simulink model "TorqueAchievedEstimationComponent"  (R2026a)
settings: Solver=FixedStepDiscrete
settings Model: DataDictionary=TractionEmotorSoftwareArchInterfaceData.sldd  Creator=dakaihu  LastModifiedBy=dakaihu

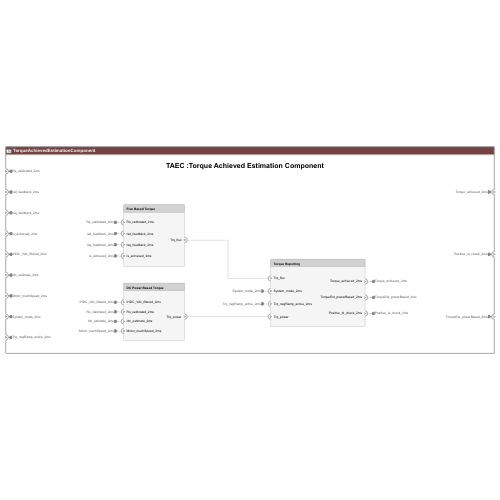
[thumbnail: Simulink's stored preview of the top-level diagram]
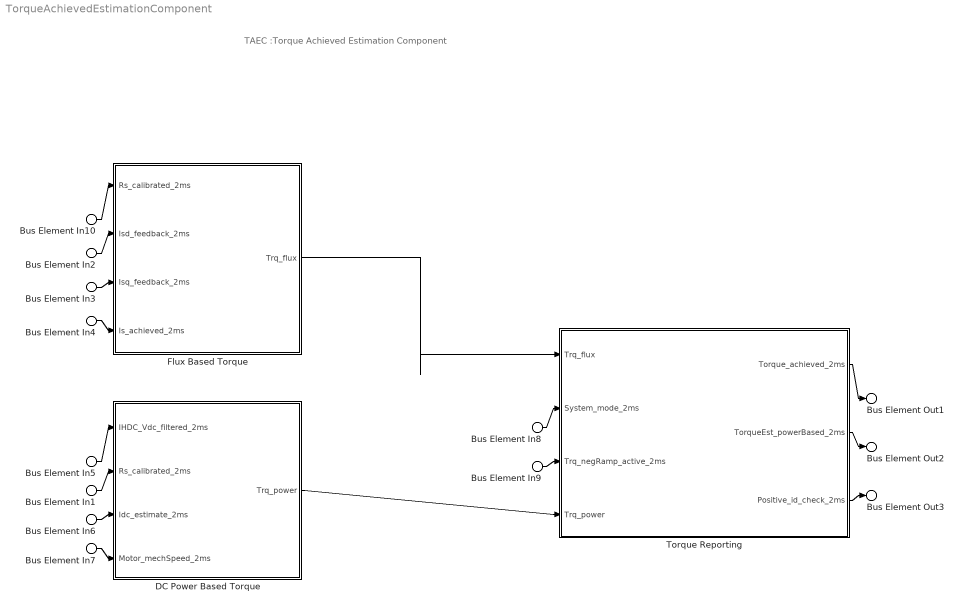
== system TorqueAchievedEstimationComponent ==
  note: TAEC :Torque Achieved Estimation Component
  Bus Element In1 : Inport  PortName=Rs_calibrated_2ms
  Bus Element In10 : Inport  PortName=Rs_calibrated_2ms
  Bus Element In2 : Inport  Port=2  PortName=Isd_feedback_2ms
  Bus Element In3 : Inport  Port=3  PortName=Isq_feedback_2ms
  Bus Element In4 : Inport  Port=4  PortName=Is_achieved_2ms
  Bus Element In5 : Inport  Port=5  PortName=IHDC_Vdc_filtered_2ms
  Bus Element In6 : Inport  Port=6  PortName=Idc_estimate_2ms
  Bus Element In7 : Inport  Port=7  PortName=Motor_mechSpeed_2ms
  Bus Element In8 : Inport  Port=8  PortName=System_mode_2ms
  Bus Element In9 : Inport  Port=9  PortName=Trq_negRamp_active_2ms
  DC Power Based Torque : Subsystem
      settings: PortSchema="{\"entries\":[{\"content\":{\"headerSize\":26,\"margin\":15,\"minimumSpacing\":25,\"sides\":[{\"content\":{\"connectorIds\":[\"In1\",\"In2\",\"In3\",\"In4\"]},\"type\":\"ConnectorPlacement.EquallySpacedRectSide\",\"uuid\":\"a0c63ab2-75fe-4bec-b2b0-6e2e00a1a5a4\"},{\"content\":{\"connectorIds\":[\"Out1\"],\"side\":\"RIGHT\"},\"type\":\"ConnectorPlacement.EquallySpacedRectSide\",\"uuid\":\"05d605ea-8968-4533-a01c-bf4aae5caa93\"},{\"content\":{\"side\":\"TOP\"},\"type\":\"ConnectorPlacement.EquallySpacedRectSide\",\"uuid\":\"27167c69-3967-4107-acce-f317c3d854af\"}]},\"type\":\"ConnectorPlacement.EquallySpacedConnector\",\"uuid\":\"c4d90da2-0f2a-4c00-bd24-85fead00d18f\"}],\"packageUris\":[\"http://schema.mathworks.com/mf0/Connector/R2020b\"],\"version\":\"1.0\"}"
  Flux Based Torque : Subsystem
      settings: PortSchema="{\"entries\":[{\"content\":{\"headerSize\":26,\"margin\":15,\"minimumSpacing\":25,\"sides\":[{\"content\":{\"connectorIds\":[\"In1\",\"In2\",\"In3\",\"In4\"]},\"type\":\"ConnectorPlacement.EquallySpacedRectSide\",\"uuid\":\"a0c63ab2-75fe-4bec-b2b0-6e2e00a1a5a4\"},{\"content\":{\"connectorIds\":[\"Out1\"],\"side\":\"RIGHT\"},\"type\":\"ConnectorPlacement.EquallySpacedRectSide\",\"uuid\":\"05d605ea-8968-4533-a01c-bf4aae5caa93\"},{\"content\":{\"side\":\"TOP\"},\"type\":\"ConnectorPlacement.EquallySpacedRectSide\",\"uuid\":\"27167c69-3967-4107-acce-f317c3d854af\"}]},\"type\":\"ConnectorPlacement.EquallySpacedConnector\",\"uuid\":\"c4d90da2-0f2a-4c00-bd24-85fead00d18f\"}],\"packageUris\":[\"http://schema.mathworks.com/mf0/Connector/R2020b\"],\"version\":\"1.0\"}"
  Torque Reporting : Subsystem
      settings: PortSchema="{\"entries\":[{\"content\":{\"headerSize\":26,\"margin\":15,\"minimumSpacing\":25,\"sides\":[{\"content\":{\"connectorIds\":[\"In1\",\"In2\",\"In4\",\"In3\"]},\"type\":\"ConnectorPlacement.EquallySpacedRectSide\",\"uuid\":\"a0c63ab2-75fe-4bec-b2b0-6e2e00a1a5a4\"},{\"content\":{\"connectorIds\":[\"Out1\",\"Out2\",\"Out3\"],\"side\":\"RIGHT\"},\"type\":\"ConnectorPlacement.EquallySpacedRectSide\",\"uuid\":\"05d605ea-8968-4533-a01c-bf4aae5caa93\"},{\"content\":{\"side\":\"TOP\"},\"type\":\"ConnectorPlacement.EquallySpacedRectSide\",\"uuid\":\"27167c69-3967-4107-acce-f317c3d854af\"}]},\"type\":\"ConnectorPlacement.EquallySpacedConnector\",\"uuid\":\"c4d90da2-0f2a-4c00-bd24-85fead00d18f\"}],\"packageUris\":[\"http://schema.mathworks.com/mf0/Connector/R2020b\"],\"version\":\"1.0\"}"
  Bus Element Out1 : Outport  PortName=Torque_achieved_2ms
  Bus Element Out3 : Outport  Port=2  PortName=Positive_id_check_2ms
  Bus Element Out2 : Outport  Port=3  PortName=TorqueEst_powerBased_2ms
  wires:
  Flux Based Torque/1(Trq_flux) -> Torque Reporting/1(Trq_flux)
  DC Power Based Torque/1(Trq_power) -> Torque Reporting/3(Trq_power)
  Torque Reporting/1(Torque_achieved_2ms) -> Bus Element Out1/1
  Torque Reporting/2(TorqueEst_powerBased_2ms) -> Bus Element Out2/1
  Bus Element In2/1 -> Flux Based Torque/2(Isd_feedback_2ms)
  Bus Element In3/1 -> Flux Based Torque/3(Isq_feedback_2ms)
  Bus Element In1/1 -> DC Power Based Torque/2(Rs_calibrated_2ms)
  Bus Element In6/1 -> DC Power Based Torque/3(Idc_estimate_2ms)
  Bus Element In7/1 -> DC Power Based Torque/4(Motor_mechSpeed_2ms)
  Bus Element In8/1 -> Torque Reporting/2(System_mode_2ms)
  Torque Reporting/3(Positive_id_check_2ms) -> Bus Element Out3/1
  Bus Element In9/1 -> Torque Reporting/4(Trq_negRamp_active_2ms)
  Bus Element In5/1 -> DC Power Based Torque/1(IHDC_Vdc_filtered_2ms)
  Bus Element In10/1 -> Flux Based Torque/1(Rs_calibrated_2ms)
  Bus Element In4/1 -> Flux Based Torque/4(Is_achieved_2ms)

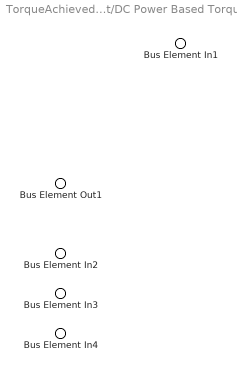
== system TorqueAchievedEstimationComponent/DC Power Based Torque ==
  Bus Element In1 : Inport  PortName=IHDC_Vdc_filtered_2ms
  Bus Element In2 : Inport  Port=2  PortName=Rs_calibrated_2ms
  Bus Element In3 : Inport  Port=3  PortName=Idc_estimate_2ms
  Bus Element In4 : Inport  Port=4  PortName=Motor_mechSpeed_2ms
  Bus Element Out1 : Outport  PortName=Trq_power

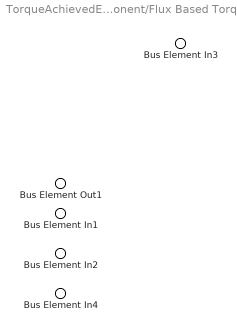
== system TorqueAchievedEstimationComponent/Flux Based Torque ==
  Bus Element In3 : Inport  PortName=Rs_calibrated_2ms
  Bus Element In1 : Inport  Port=2  PortName=Isd_feedback_2ms
  Bus Element In2 : Inport  Port=3  PortName=Isq_feedback_2ms
  Bus Element In4 : Inport  Port=4  PortName=Is_achieved_2ms
  Bus Element Out1 : Outport  PortName=Trq_flux

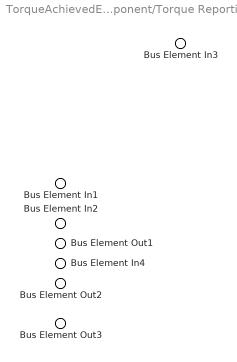
== system TorqueAchievedEstimationComponent/Torque Reporting ==
  Bus Element In1 : Inport  PortName=Trq_flux
  Bus Element In3 : Inport  Port=2  PortName=System_mode_2ms
  Bus Element In2 : Inport  Port=3  PortName=Trq_power
  Bus Element In4 : Inport  Port=4  PortName=Trq_negRamp_active_2ms
  Bus Element Out1 : Outport  PortName=Torque_achieved_2ms
  Bus Element Out2 : Outport  Port=2  PortName=TorqueEst_powerBased_2ms
  Bus Element Out3 : Outport  Port=3  PortName=Positive_id_check_2ms
